simulink model "Test_System"  (R2024b)
settings: Solver=VariableStepAuto  StartTime=0.0  StopTime=10.0  RelTol=1e-3
settings Model: Creator=sabpi  LastModifiedBy=sabpi

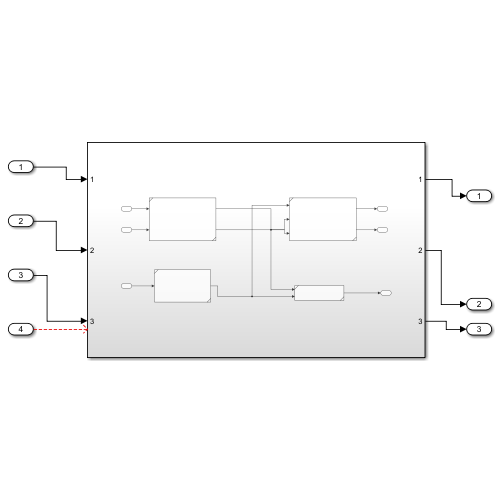
[thumbnail: Simulink's stored preview of the top-level diagram]
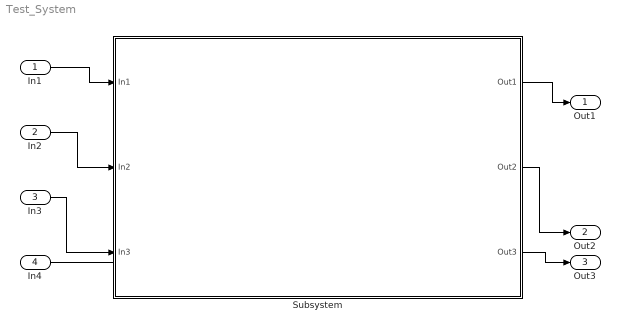
== system Test_System ==
  In1 : Inport
  In2 : Inport  Port=2
  In3 : Inport  Port=3
  In4 : Inport  Port=4
  Subsystem : Subsystem
  Out1 : Outport
  Out2 : Outport  Port=2
  Out3 : Outport  Port=3
  wires:
  In1/1 -> Subsystem/1(In1)
  In2/1 -> Subsystem/2(In2)
  In3/1 -> Subsystem/3(In3)
  In4/1 -> ?
  Subsystem/1(Out1) -> Out1/1
  Subsystem/2(Out2) -> Out2/1
  Subsystem/3(Out3) -> Out3/1

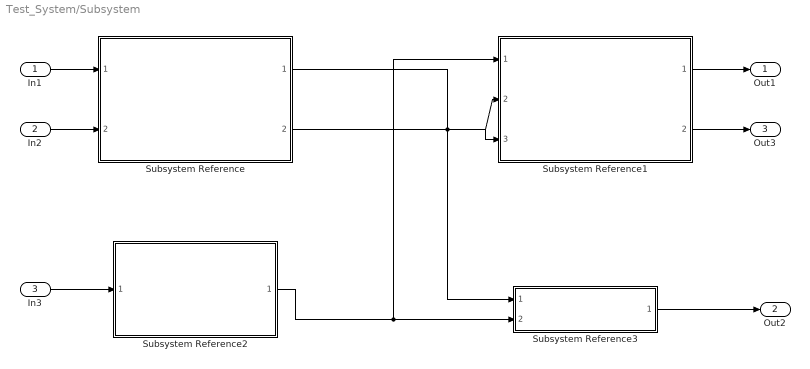
== system Test_System/Subsystem ==
  In1 : Inport
  In2 : Inport  Port=2
  In3 : Inport  Port=3
  Subsystem Reference : Subsystem  ReferencedSubsystem=Prova_1
  Subsystem Reference1 : Subsystem  ReferencedSubsystem=Prova_2
  Subsystem Reference2 : Subsystem  ReferencedSubsystem=Prova_3
  Subsystem Reference3 : Subsystem  ReferencedSubsystem=Prova_4
  Out1 : Outport
  Out2 : Outport  Port=2
  Out3 : Outport  Port=3
  wires:
  Subsystem Reference2/1 -> Subsystem Reference3/2, Subsystem Reference1/1
  Subsystem Reference/1 -> Subsystem Reference3/1, Subsystem Reference1/2
  In1/1 -> Subsystem Reference/1
  In2/1 -> Subsystem Reference/2
  In3/1 -> Subsystem Reference2/1
  Subsystem Reference1/1 -> Out1/1
  Subsystem Reference3/1 -> Out2/1
  Subsystem Reference/2 -> Subsystem Reference1/3
  Subsystem Reference1/2 -> Out3/1
